simulink model "test_mdl"  (R2018b)
settings: Solver=FixedStepDiscrete  StartTime=0.0  StopTime=20.0  FixedStep=0.2  RelTol=1e-3
undefined symbols (not defined in the file): A, B, C, m, n, T, x0
settings Model: Creator=bradyplanden  LastModifiedBy=bradyplanden
settings OptimizationCC: DefaultParameterBehavior=Inlined
settings SFSimCC: SimCustomHeaderCode="#include \"fmpc.h\""  SimUserSources=fmpc_simulink.c  SimUserIncludeDirs=/usr/lib  SimUserLibraries=libblas.dylib liblapack.dylib  SimUseLocalCustomCode=off  SimAnalyzeCustomCode=on
settings RTWCC: GenerateReport=on  RTWUseLocalCustomCode=off  RTWUseSimCustomCode=on  CustomHeaderCode="#include \"fmpc.h\""  CustomInclude=/usr/lib  CustomSource=fmpc_simulink.c  CustomLibrary=libblas.dylib liblapack.dylib  LaunchReport=on
settings CodeAppCC: ForceParamTrailComments=on  StateflowObjectComments=on  MATLABSourceComments=on
settings GRTTargetCC: TargetLangStandard=C89/C90 (ANSI)

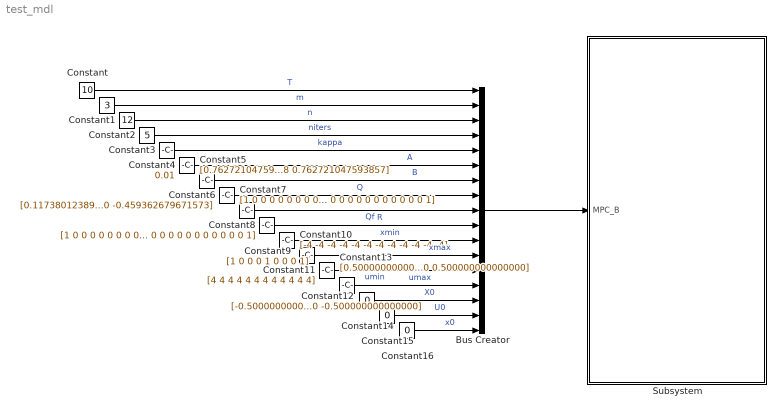
== system test_mdl ==
  Bus Creator : BusCreator  Inputs=17
  Constant : Constant  Value=10  SampleTime=-1
  Constant1 : Constant  Value=3  SampleTime=-1
  Constant10 : Constant  Value=|  SampleTime=-1
      | [-4
      | -4
      | -4
      | -4
      | -4
      | -4
      | -4
      | -4
      | -4
      | -4
      | -4
      | -4]
  Constant11 : Constant  Value=|  SampleTime=-1
      | [4
      | 4
      | 4
      | 4
      | 4
      | 4
      | 4
      | 4
      | 4
      | 4
      | 4
      | 4]
  Constant12 : Constant  Value=|  SampleTime=-1
      | [-0.500000000000000
      | -0.500000000000000
      | -0.500000000000000]
  Constant13 : Constant  Value=|  SampleTime=-1
      | [0.500000000000000
      | 0.500000000000000
      | 0.500000000000000]
  Constant14 : Constant  Value=0  SampleTime=-1
  Constant15 : Constant  Value=0  SampleTime=-1
  Constant16 : Constant  Value=0  SampleTime=-1
  Constant2 : Constant  Value=12  OutDataTypeStr=int8  SampleTime=-1
  Constant3 : Constant  Value=5  SampleTime=-1
  Constant4 : Constant  Value=0.01  SampleTime=-1
  Constant5 : Constant  Value=|  SampleTime=-1
      | [0.762721047593857	0.114882546593898	0.00247654474066823	2.09380749408769e-05	9.42229417535085e-08	2.63060135287668e-10	0.459613939727602	0.0198131117128797	0.000251260056028671	1.50757506761672e-06	5.26123024735364e-09	1.19993006342024e-11
      | 0.114882546593898	0.765197592334525	0.114903484668839	0.00247663896360998	2.09383380010122e-05	9.42229417535096e-08	0.0198131117128796	0.459865199783630	0.0198146192879473	0.000251265317258919	1.50758706691736e-06	5.26123024735407e-09
      | 0.00247654474066823	0.114903484668839	0.765197686557466	0.114903484931899	0.00247663896360999	2.09380749408770e-05	0.000251260056028671	0.0198146192879473	0.459865205044861	0.0198146192999466	0.000251265317258919	1.50757506761673e-06
      | 2.09380749408769e-05	0.00247663896360998	0.114903484931899	0.765197686557467	0.114903484668839	0.00247654474066823	1.50757506761672e-06	0.000251265317258918	0.0198146192999466	0.459865205044861	0.0198146192879473	0.000251260056028672
      | 9.42229417535087e-08	2.09383380010122e-05	0.00247663896360998	0.114903484668839	0.765197592334525	0.114882546593898	5.26123024735378e-09	1.50758706691736e-06	0.000251265317258919	0.0198146192879473	0.459865199783631	0.0198131117128796
      | 2.63060135287738e-10	9.42229417535093e-08	2.09380749408769e-05	0.00247654474066823	0.114882546593898	0.762721047593857	1.19993006342118e-11	5.26123024735394e-09	1.50757506761673e-06	0.000251260056028671	0.0198131117128797	0.459613939727602
      | -0.899414767742325	0.420238976357871	0.0193120991758899	0.000248250167123685	1.49706460642265e-06	5.23723164608530e-09	0.762721047593857	0.114882546593898	0.00247654474066823	2.09380749408769e-05	9.42229417535083e-08	2.63060135287700e-10
      | 0.420238976357871	-0.880102668566434	0.420487226524995	0.0193135962404963	0.000248255404355332	1.49706460642266e-06	0.114882546593898	0.765197592334525	0.114903484668839	0.00247663896360998	2.09383380010123e-05	9.42229417535099e-08
      | 0.0193120991758899	0.420487226524995	-0.880101171501828	0.420487231762227	0.0193135962404964	0.000248250167123686	0.00247654474066823	0.114903484668839	0.765197686557467	0.114903484931899	0.00247663896360999	2.09380749408770e-05
      | 0.000248250167123685	0.0193135962404963	0.420487231762227	-0.880101171501828	0.420487226524995	0.0193120991758899	2.09380749408769e-05	0.00247663896360998	0.114903484931899	0.765197686557467	0.114903484668839	0.00247654474066823
      | 1.49706460642265e-06	0.000248255404355331	0.0193135962404963	0.420487226524995	-0.880102668566434	0.420238976357871	9.42229417535088e-08	2.09383380010122e-05	0.00247663896360998	0.114903484668839	0.765197592334525	0.114882546593898
      | 5.23723164608547e-09	1.49706460642265e-06	0.000248250167123685	0.0193120991758899	0.420238976357872	-0.899414767742325	2.63060135287715e-10	9.42229417535098e-08	2.09380749408769e-05	0.00247654474066823	0.114882546593898	0.762721047593857]
  Constant6 : Constant  Value=|  SampleTime=-1
      | [0.117380123896011	2.11270479473799e-05	9.47500646873726e-08
      | -0.117401251208020	0.00251870461362123	2.11273120101163e-05
      | -0.00249767205267819	0.119898828510133	0.00251870461462378
      | -2.10328255067807e-05	5.01412713432847e-13	0.119898828774196
      | -9.44870044752643e-08	-0.119898828246070	9.47505659474636e-08
      | -2.63561428521144e-10	-0.00251860986355638	-0.119877701198123
      | 0.439800828014722	0.000251254794798423	1.50756306831608e-06
      | -0.440052088070751	0.0198131117008803	0.000251260056028671
      | -0.0195633592319186	0.459613939727602	0.0198131117248790
      | -0.000249757742191302	1.19993147362774e-11	0.459613944988832
      | -1.50232583667001e-06	-0.459613934466372	1.50757506762675e-06
      | -5.24923094671973e-09	-0.0198116041378120	-0.459362679671573]
  Constant7 : Constant  Value=|  SampleTime=-1
      | [1	0	0	0	0	0	0	0	0	0	0	0
      | 0	1	0	0	0	0	0	0	0	0	0	0
      | 0	0	1	0	0	0	0	0	0	0	0	0
      | 0	0	0	1	0	0	0	0	0	0	0	0
      | 0	0	0	0	1	0	0	0	0	0	0	0
      | 0	0	0	0	0	1	0	0	0	0	0	0
      | 0	0	0	0	0	0	1	0	0	0	0	0
      | 0	0	0	0	0	0	0	1	0	0	0	0
      | 0	0	0	0	0	0	0	0	1	0	0	0
      | 0	0	0	0	0	0	0	0	0	1	0	0
      | 0	0	0	0	0	0	0	0	0	0	1	0
      | 0	0	0	0	0	0	0	0	0	0	0	1]
  Constant8 : Constant  Value=|  SampleTime=-1
      | [1	0	0	0	0	0	0	0	0	0	0	0
      | 0	1	0	0	0	0	0	0	0	0	0	0
      | 0	0	1	0	0	0	0	0	0	0	0	0
      | 0	0	0	1	0	0	0	0	0	0	0	0
      | 0	0	0	0	1	0	0	0	0	0	0	0
      | 0	0	0	0	0	1	0	0	0	0	0	0
      | 0	0	0	0	0	0	1	0	0	0	0	0
      | 0	0	0	0	0	0	0	1	0	0	0	0
      | 0	0	0	0	0	0	0	0	1	0	0	0
      | 0	0	0	0	0	0	0	0	0	1	0	0
      | 0	0	0	0	0	0	0	0	0	0	1	0
      | 0	0	0	0	0	0	0	0	0	0	0	1]
  Constant9 : Constant  Value=|  SampleTime=-1
      | [1	0	0
      | 0	1	0
      | 0	0	1]
  Subsystem : Subsystem
  wires:
  Constant/1 -> Bus Creator/1  "T"
  Bus Creator/1 -> Subsystem/1(MPC_B)
  Constant1/1 -> Bus Creator/2  "m"
  Constant2/1 -> Bus Creator/3  "n"
  Constant3/1 -> Bus Creator/4  "niters"
  Constant4/1 -> Bus Creator/5  "kappa"
  Constant15/1 -> Bus Creator/16  "U0"
  Constant16/1 -> Bus Creator/17  "x0"
  Constant8/1 -> Bus Creator/9  "Qf"
  Constant5/1 -> Bus Creator/6  "A"
  Constant6/1 -> Bus Creator/7  "B"
  Constant7/1 -> Bus Creator/8  "Q"
  Constant13/1 -> Bus Creator/14  "umax"
  Constant12/1 -> Bus Creator/13  "umin"
  Constant11/1 -> Bus Creator/12  "xmax"
  Constant10/1 -> Bus Creator/11  "xmin"
  Constant9/1 -> Bus Creator/10  "R"
  Constant14/1 -> Bus Creator/15  "X0"

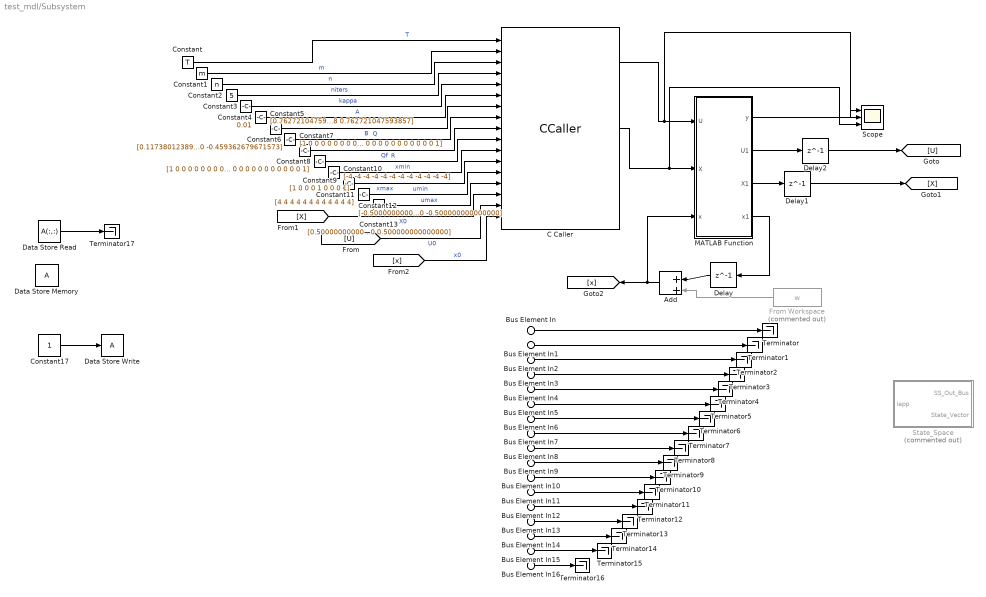
== system test_mdl/Subsystem ==
  Bus Element In : Inport  PortName=MPC_B  Element=T
  Bus Element In1 : Inport  PortName=MPC_B  Element=m
  Bus Element In2 : Inport  PortName=MPC_B  Element=n
  Bus Element In3 : Inport  PortName=MPC_B  Element=niters
  Bus Element In4 : Inport  PortName=MPC_B  Element=kappa
  Bus Element In5 : Inport  PortName=MPC_B  Element=A
  Bus Element In6 : Inport  PortName=MPC_B  Element=B
  Bus Element In7 : Inport  PortName=MPC_B  Element=Q
  Bus Element In8 : Inport  PortName=MPC_B  Element=Qf
  Bus Element In9 : Inport  PortName=MPC_B  Element=R
  Bus Element In10 : Inport  PortName=MPC_B  Element=xmin
  Bus Element In11 : Inport  PortName=MPC_B  Element=xmax
  Bus Element In12 : Inport  PortName=MPC_B  Element=umin
  Bus Element In13 : Inport  PortName=MPC_B  Element=umax
  Bus Element In14 : Inport  PortName=MPC_B  Element=X0
  Bus Element In15 : Inport  PortName=MPC_B  Element=U0
  Bus Element In16 : Inport  PortName=MPC_B  Element=x0
  Add : Sum  Inputs=+|+
  C Caller : CCaller  FunctionName=mpc  PortSpecificationStruct="%)30     .    P!P   8    (     @         %    \"    !0    !     0         %  0 \"0    $    V    07)G3F%M90  4&]R=$YA;64 4V-O<&4     26YD97@     5'EP90      4VEZ90         .    ,     8    (    !          %    \"     $    #     0         0  , ;W5T  X    P    !@    @    $          4    (     0    ,    !         !   P!O=70 #@   #@    &    \"     0         !0    @    !    !@    $         $     8   !/=7 ...(+9546 chars)"
  Constant : Constant  Value=T  OutDataTypeStr=Inherit: Inherit via back propagation  SampleTime=-1
  Constant1 : Constant  Value=m  OutDataTypeStr=Inherit: Inherit via back propagation  SampleTime=-1
  Constant10 : Constant  Value=|  OutDataTypeStr=Inherit: Inherit via back propagation  SampleTime=-1
      | [-4
      | -4
      | -4
      | -4
      | -4
      | -4
      | -4
      | -4
      | -4
      | -4
      | -4
      | -4]
  Constant11 : Constant  Value=|  OutDataTypeStr=Inherit: Inherit via back propagation  SampleTime=-1
      | [4
      | 4
      | 4
      | 4
      | 4
      | 4
      | 4
      | 4
      | 4
      | 4
      | 4
      | 4]
  Constant12 : Constant  Value=|  OutDataTypeStr=Inherit: Inherit via back propagation  SampleTime=-1
      | [-0.500000000000000
      | -0.500000000000000
      | -0.500000000000000]
  Constant13 : Constant  Value=|  OutDataTypeStr=Inherit: Inherit via back propagation  SampleTime=-1
      | [0.500000000000000
      | 0.500000000000000
      | 0.500000000000000]
  Constant17 : Constant
  Constant2 : Constant  Value=n  OutDataTypeStr=Inherit: Inherit via back propagation  SampleTime=-1
  Constant3 : Constant  Value=5  OutDataTypeStr=Inherit: Inherit via back propagation  SampleTime=-1
  Constant4 : Constant  Value=0.01  OutDataTypeStr=Inherit: Inherit via back propagation  SampleTime=-1
  Constant5 : Constant  Value=|  OutDataTypeStr=Inherit: Inherit via back propagation  SampleTime=-1
      | [0.762721047593857	0.114882546593898	0.00247654474066823	2.09380749408769e-05	9.42229417535085e-08	2.63060135287668e-10	0.459613939727602	0.0198131117128797	0.000251260056028671	1.50757506761672e-06	5.26123024735364e-09	1.19993006342024e-11
      | 0.114882546593898	0.765197592334525	0.114903484668839	0.00247663896360998	2.09383380010122e-05	9.42229417535096e-08	0.0198131117128796	0.459865199783630	0.0198146192879473	0.000251265317258919	1.50758706691736e-06	5.26123024735407e-09
      | 0.00247654474066823	0.114903484668839	0.765197686557466	0.114903484931899	0.00247663896360999	2.09380749408770e-05	0.000251260056028671	0.0198146192879473	0.459865205044861	0.0198146192999466	0.000251265317258919	1.50757506761673e-06
      | 2.09380749408769e-05	0.00247663896360998	0.114903484931899	0.765197686557467	0.114903484668839	0.00247654474066823	1.50757506761672e-06	0.000251265317258918	0.0198146192999466	0.459865205044861	0.0198146192879473	0.000251260056028672
      | 9.42229417535087e-08	2.09383380010122e-05	0.00247663896360998	0.114903484668839	0.765197592334525	0.114882546593898	5.26123024735378e-09	1.50758706691736e-06	0.000251265317258919	0.0198146192879473	0.459865199783631	0.0198131117128796
      | 2.63060135287738e-10	9.42229417535093e-08	2.09380749408769e-05	0.00247654474066823	0.114882546593898	0.762721047593857	1.19993006342118e-11	5.26123024735394e-09	1.50757506761673e-06	0.000251260056028671	0.0198131117128797	0.459613939727602
      | -0.899414767742325	0.420238976357871	0.0193120991758899	0.000248250167123685	1.49706460642265e-06	5.23723164608530e-09	0.762721047593857	0.114882546593898	0.00247654474066823	2.09380749408769e-05	9.42229417535083e-08	2.63060135287700e-10
      | 0.420238976357871	-0.880102668566434	0.420487226524995	0.0193135962404963	0.000248255404355332	1.49706460642266e-06	0.114882546593898	0.765197592334525	0.114903484668839	0.00247663896360998	2.09383380010123e-05	9.42229417535099e-08
      | 0.0193120991758899	0.420487226524995	-0.880101171501828	0.420487231762227	0.0193135962404964	0.000248250167123686	0.00247654474066823	0.114903484668839	0.765197686557467	0.114903484931899	0.00247663896360999	2.09380749408770e-05
      | 0.000248250167123685	0.0193135962404963	0.420487231762227	-0.880101171501828	0.420487226524995	0.0193120991758899	2.09380749408769e-05	0.00247663896360998	0.114903484931899	0.765197686557467	0.114903484668839	0.00247654474066823
      | 1.49706460642265e-06	0.000248255404355331	0.0193135962404963	0.420487226524995	-0.880102668566434	0.420238976357871	9.42229417535088e-08	2.09383380010122e-05	0.00247663896360998	0.114903484668839	0.765197592334525	0.114882546593898
      | 5.23723164608547e-09	1.49706460642265e-06	0.000248250167123685	0.0193120991758899	0.420238976357872	-0.899414767742325	2.63060135287715e-10	9.42229417535098e-08	2.09380749408769e-05	0.00247654474066823	0.114882546593898	0.762721047593857]
  Constant6 : Constant  Value=|  OutDataTypeStr=Inherit: Inherit via back propagation  SampleTime=-1
      | [0.117380123896011	2.11270479473799e-05	9.47500646873726e-08
      | -0.117401251208020	0.00251870461362123	2.11273120101163e-05
      | -0.00249767205267819	0.119898828510133	0.00251870461462378
      | -2.10328255067807e-05	5.01412713432847e-13	0.119898828774196
      | -9.44870044752643e-08	-0.119898828246070	9.47505659474636e-08
      | -2.63561428521144e-10	-0.00251860986355638	-0.119877701198123
      | 0.439800828014722	0.000251254794798423	1.50756306831608e-06
      | -0.440052088070751	0.0198131117008803	0.000251260056028671
      | -0.0195633592319186	0.459613939727602	0.0198131117248790
      | -0.000249757742191302	1.19993147362774e-11	0.459613944988832
      | -1.50232583667001e-06	-0.459613934466372	1.50757506762675e-06
      | -5.24923094671973e-09	-0.0198116041378120	-0.459362679671573]
  Constant7 : Constant  Value=|  OutDataTypeStr=Inherit: Inherit via back propagation  SampleTime=-1
      | [1	0	0	0	0	0	0	0	0	0	0	0
      | 0	1	0	0	0	0	0	0	0	0	0	0
      | 0	0	1	0	0	0	0	0	0	0	0	0
      | 0	0	0	1	0	0	0	0	0	0	0	0
      | 0	0	0	0	1	0	0	0	0	0	0	0
      | 0	0	0	0	0	1	0	0	0	0	0	0
      | 0	0	0	0	0	0	1	0	0	0	0	0
      | 0	0	0	0	0	0	0	1	0	0	0	0
      | 0	0	0	0	0	0	0	0	1	0	0	0
      | 0	0	0	0	0	0	0	0	0	1	0	0
      | 0	0	0	0	0	0	0	0	0	0	1	0
      | 0	0	0	0	0	0	0	0	0	0	0	1]
  Constant8 : Constant  Value=|  OutDataTypeStr=Inherit: Inherit via back propagation  SampleTime=-1
      | [1	0	0	0	0	0	0	0	0	0	0	0
      | 0	1	0	0	0	0	0	0	0	0	0	0
      | 0	0	1	0	0	0	0	0	0	0	0	0
      | 0	0	0	1	0	0	0	0	0	0	0	0
      | 0	0	0	0	1	0	0	0	0	0	0	0
      | 0	0	0	0	0	1	0	0	0	0	0	0
      | 0	0	0	0	0	0	1	0	0	0	0	0
      | 0	0	0	0	0	0	0	1	0	0	0	0
      | 0	0	0	0	0	0	0	0	1	0	0	0
      | 0	0	0	0	0	0	0	0	0	1	0	0
      | 0	0	0	0	0	0	0	0	0	0	1	0
      | 0	0	0	0	0	0	0	0	0	0	0	1]
  Constant9 : Constant  Value=|  OutDataTypeStr=Inherit: Inherit via back propagation  SampleTime=-1
      | [1	0	0
      | 0	1	0
      | 0	0	1]
  Data Store Memory : DataStoreMemory  ReadBeforeWriteMsg=warning  WriteAfterWriteMsg=warning  WriteAfterReadMsg=warning  VectorParams1D=off  ShowAdditionalParam=off
      settings: LockScale=on
  Data Store Read : DataStoreRead  DataStoreElements=A(:,:)
  Data Store Write : DataStoreWrite  DataStoreElements=A
  Delay : Delay  DelayLength=1  InitialCondition=x0
  Delay1 : Delay  DelayLength=1  InitialCondition=zeros(n,T)
  Delay2 : Delay  DelayLength=1  InitialCondition=zeros(m,T)  InputProcessing=Inherited
  From Workspace : FromWorkspace  Commented=on  VariableName=w  SampleTime=0.2  OutputAfterFinalValue=Setting to zero
  MATLAB Function : MATLAB Function  TreatAsAtomicUnit=on
  Scope : Scope  NumInputPorts=3
  State_Space : Subsystem  Commented=on
  Terminator{,1..17} (18 alike) : Terminator
  wires:
  Bus Element In/1 -> Terminator/1
  Bus Element In1/1 -> Terminator1/1
  Bus Element In2/1 -> Terminator2/1
  Bus Element In3/1 -> Terminator3/1
  Bus Element In4/1 -> Terminator4/1
  Bus Element In5/1 -> Terminator5/1
  Bus Element In6/1 -> Terminator6/1
  Bus Element In7/1 -> Terminator7/1
  Bus Element In8/1 -> Terminator8/1
  Bus Element In9/1 -> Terminator9/1
  Bus Element In10/1 -> Terminator10/1
  Bus Element In11/1 -> Terminator11/1
  Bus Element In12/1 -> Terminator12/1
  Bus Element In13/1 -> Terminator13/1
  Bus Element In14/1 -> Terminator14/1
  Bus Element In15/1 -> Terminator15/1
  Bus Element In16/1 -> Terminator16/1
  Constant17/1 -> Data Store Write/1
  Data Store Read/1 -> Terminator17/1
  MATLAB Function/4(x1) -> Delay/1
  Delay/1 -> Add/1
  MATLAB Function/2(U1) -> Delay2/1
  MATLAB Function/3(X1) -> Delay1/1
  MATLAB Function/1(y) -> Scope/1
  Delay1/1 -> [X]
  Delay2/1 -> [U]
  From Workspace/1 -> Add/2
  Add/1 -> MATLAB Function/3(x), [x]
  C Caller/1 -> Scope/2, MATLAB Function/1(U)
  C Caller/2 -> Scope/3, MATLAB Function/2(X)
  [x] -> C Caller/17  "x0"
  Constant13/1 -> C Caller/14  "umax"
  Constant12/1 -> C Caller/13  "umin"
  [U] -> C Caller/16  "U0"
  Constant11/1 -> C Caller/12  "xmax"
  Constant10/1 -> C Caller/11  "xmin"
  [X] -> C Caller/15  "X0"
  Constant9/1 -> C Caller/10  "R"
  Constant8/1 -> C Caller/9  "Qf"
  Constant7/1 -> C Caller/8  "Q"
  Constant6/1 -> C Caller/7  "B"
  Constant5/1 -> C Caller/6  "A"
  Constant4/1 -> C Caller/5  "kappa"
  Constant3/1 -> C Caller/4  "niters"
  Constant2/1 -> C Caller/3  "n"
  Constant1/1 -> C Caller/2  "m"
  Constant/1 -> C Caller/1  "T"

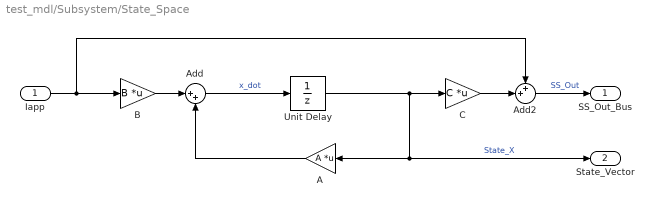
== system test_mdl/Subsystem/State_Space ==
  Iapp : Inport
  A : Gain  Gain=A  Multiplication=Matrix(K*u)
  Add : Sum  Inputs=|++
  Add2 : Sum  Inputs=++|
  B : Gain  Gain=B  Multiplication=Matrix(K*u)
  C : Gain  Gain=C  Multiplication=Matrix(K*u)
  Unit Delay : UnitDelay  SampleTime=-1
  SS_Out_Bus : Outport
  State_Vector : Outport  Port=2
  wires:
  Unit Delay/1 -> State_Vector/1, A/1, C/1  "State_X"
  B/1 -> Add/1
  Add/1 -> Unit Delay/1  "x_dot"
  C/1 -> Add2/2
  A/1 -> Add/2
  Iapp/1 -> Add2/1, B/1
  Add2/1 -> SS_Out_Bus/1  "SS_Out"

== matlab function test_mdl/Subsystem/MATLAB Function ==
  data: U input; y output; U1 output; X1 output; X input; x input; x1 output; A parameter; T parameter; B parameter; n parameter; m parameter; x0 parameter
function [y,U1,X1,x1] = fcn(U,X,x, A, T, B, n, m, x0)
u = U(:,1);

x1 =A*x+B*u;
X1 = [X(:,2:10),zeros(12,1)];
U1 = [U(:,2:10),zeros(3,1)];

y = u;
